simulink model "Baseband_LDPC_BPSK_MULTIPATH"  (R2017b)
settings: Solver=FixedStepDiscrete  StartTime=0.0  StopTime=20  RelTol=1e-3
undefined symbols (not defined in the file or in its folder): dvbs2ldpc
libraries: commchan3 x2, commdigbbndpm3 x2, commblkcod2 x2, commsink2 x1, commrandsrc3 x1
settings Model: Creator=m.s  LastModifiedBy=m.s

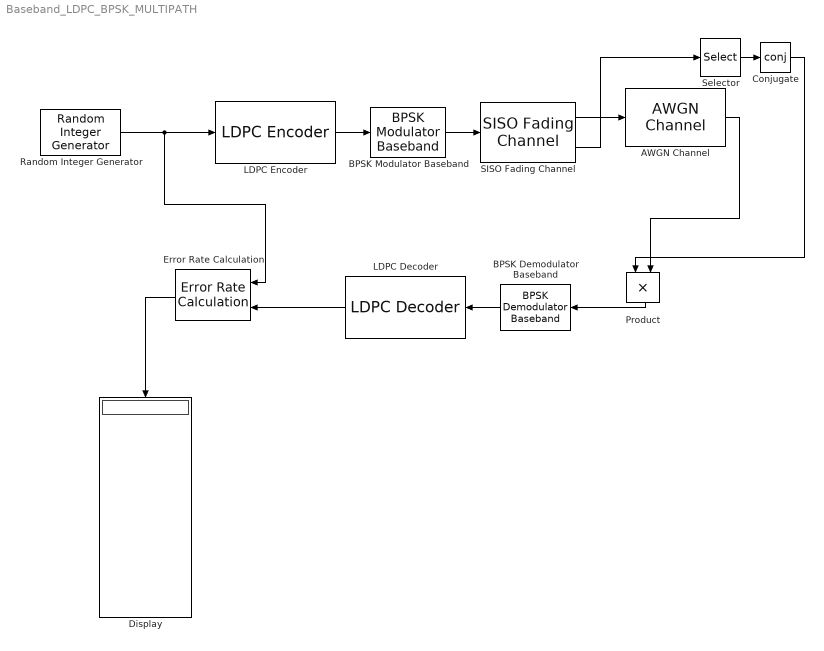
== system Baseband_LDPC_BPSK_MULTIPATH ==
  AWGN Channel : commchan3/AWGN Channel  InputProcessing=Columns as channels (frame based)  seed=67  noiseMode="Signal to noise ratio  (SNR)"  EbNodB=10  EsNodB=10  SNRdB=0  bitsPerSym=1  Ps=1  Tsym=1  variance=1
  BPSK Demodulator Baseband : commdigbbndpm3/BPSK Demodulator Baseband  DecType=Log-likelihood ratio  VarSource=Dialog  Variance=1  Ph=0  outDtype=double  derotateFactorWordLen=16  derotateFactorDataTypeStr=Inherit: Same word length as input  derotateFactorLastDataTypeStr=Inherit: Same word length as input
  BPSK Modulator Baseband : commdigbbndpm3/BPSK Modulator Baseband  Ph=0  outDtype=double  outWordLen=16  outUDDataType=sfix(16)  outFracLenMode=Best precision  outFracLen=15  outDataTypeStr=double  outLastDataTypeStr=double
  Conjugate : Math  Operator=conj  RndMeth=Zero  SaturateOnIntegerOverflow=on
  Display : Display
  Error Rate Calculation : commsink2/Error Rate Calculation  N=0  st_delay=0  cp_mode=Entire frame  subframe=[]  PMode=Port  WsName=ErrorVec  RsMode2=off  stop=off  numErr=100  maxBits=1e6
  LDPC Decoder : commblkcod2/LDPC Decoder  ParityCheckMat=dvbs2ldpc(1/2)  OutputFmt=Information part  DecisionType=Hard decision  OutputDataType=double  NumIter=50  DoParityCheck=off  OutputNumIter=off  OutputFinalChecks=off
      settings: SourceProductName=Communications System Toolbox  SourceProductBaseCode=CM
  LDPC Encoder : commblkcod2/LDPC Encoder  ParityCheckMat=dvbs2ldpc(1/2)
      settings: SourceProductName=Communications System Toolbox  SourceProductBaseCode=CM
  Product : Product
  Random Integer Generator : commrandsrc3/Random Integer Generator  SetSize=2  SeedSource=Parameter  Seed=0  SampleTime=1e-4  SamplesPerFrame=32400  OutputDataType=double  SimulateUsing=Interpreted execution
  SISO Fading Channel : commchan3/SISO Fading Channel  PathDelays=[0 2e-4 4e-4]  AveragePathGains=[0 -3 -6]  NormalizePathGains=on  FadingDistribution=Rayleigh  KFactor=3  DirectPathDopplerShift=0  DirectPathInitialPhase=0  MaximumDopplerShift=30  DopplerSpectrum=ds  RandomStream=mt19937ar with seed  RandomNumGenerator=mt19937ar  Seed=73  PathGainsOutputPort=on  ChannelFilterDelayOutputPort=off  SimulateUsing=Interpreted execution  Visualization=Off  PathsForDopplerDisplay=1  SamplesToDisplay=25%
      settings: SourceProductName=Communications System Toolbox
  Selector : Selector  NumberOfDimensions=2  InputPortWidth=3  IndexOptions=Select all,Index vector (dialog)  Indices=[1 3],1  OutputSizes=1,1
  wires:
  Error Rate Calculation/1 -> Display/1
  Random Integer Generator/1 -> Error Rate Calculation/1, LDPC Encoder/1
  LDPC Encoder/1 -> BPSK Modulator Baseband/1
  LDPC Decoder/1 -> Error Rate Calculation/2
  BPSK Demodulator Baseband/1 -> LDPC Decoder/1
  BPSK Modulator Baseband/1 -> SISO Fading Channel/1
  SISO Fading Channel/2 -> Selector/1
  Selector/1 -> Conjugate/1
  SISO Fading Channel/1 -> AWGN Channel/1
  Conjugate/1 -> Product/1
  AWGN Channel/1 -> Product/2
  Product/1 -> BPSK Demodulator Baseband/1
